simulink model "base"  (Simulink 7.2)
settings: Solver=FixedStepDiscrete  StartTime=0.0  StopTime=inf  FixedStep=0.001  RelTol=1e-3
PostLoadFcn:
  | , if any(exist('dsrtsu_mdlpostloadfcn', 'file') == [2, 3, 6]), try dsrtsu_mdlpostloadfcn('Execute', bdroot); catch fprintf('Error in PostLoadFcn (dsrtsu_mdlpostloadfcn) for model "%s":\n %s\n', bdroot, lasterr); end, end,
InitFcn:
  | DS4504_InitCallback(bdroot);
undefined symbols (not defined in the file or in its folder): IP, UDP
libraries: ds4504base_library x4, dsextras x1
settings Model: DSRTSU_INTERNAL_RTI_VER=340  DSRTSU_INTERNAL_RTI_TYPE=rti1005  Creator=yamakawa  LastModifiedBy=higo
settings OptimizationCC: BlockReduction=off  InlineInvariantSignals=on  InitFltsAndDblsToZero=on
settings DebuggingCC: SaveWithParameterizedLinksMsg=none  SignalResolutionControl=TryResolveAllWithWarning  MultiTaskDSMMsg=warning  MultiTaskCondExecSysMsg=none  StrictBusMsg=None
settings HardwareCC: ProdIntDivRoundTo=Zero  ProdEndianess=BigEndian  ProdHWDeviceType=Specified  TargetIntDivRoundTo=Zero  TargetEndianess=BigEndian
settings RTWCC: SystemTargetFile=rti1005.tlc  MakeCommand=make_rti  TemplateMakefile=rti1005.tmf  Description=dSPACE DS1005 Hardware Platform  ProcessScript=rti1005_make_rtw_hook  IncludeERTFirstTime=on
settings STFCustomTargetCC: TargetFcnLib=ansi_tfl_tmw.mat  SystemTargetFile=rti1005.tlc
settings GRTTargetCC: TargetFcnLib=ansi_tfl_tmw.mat  CompOptLevelCompliant=off  MatFileLogging=off  ExtModeMexFile=noextcomm
settings CustomProperty: DataType=RTWOptions_EnumType_C__dSPACE_matlab_rti1005_tlc_rti1005_InitialSimState  Value=STOP
settings EnumStrPairs: String=RUN

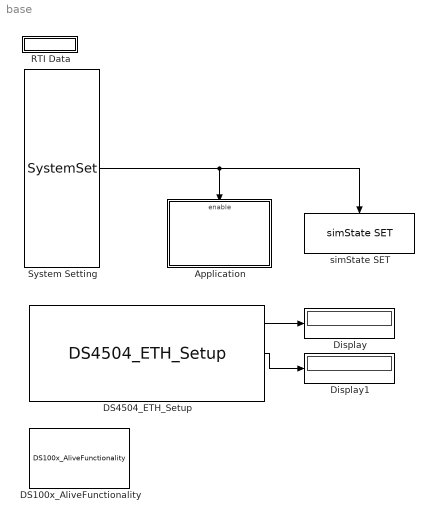
== system base ==
  Application : Subsystem  TreatAsAtomicUnit=on
  DS100x_AliveFunctionality : ds4504base_library/DS100x_AliveFunctionality  SystemSampleTime=-1  boardID=1
  DS4504_ETH_Setup : ds4504base_library/DS4504_ETH_Setup  boardID=1  IP=167888051  SM=4294901760  detectIP=off  numberApps=1  appTypes=1  appModes=1  generallyAcceptAnyIP=on  useChecksum=on  QNXSchedulerTimeInterval=50  receiveTimerPeriod=1  watchdogTimeoutSteps=10  rebootDS4504=on  DisplayMessages=on  ShowDialogBox=on  IP_String=10.1.196.179  warning1=on  warning2=on  warning3=on  warning4=on  warning5=on  disable_check=off
  Display : Display
  Display1 : Display
  RTI Data : Subsystem  Tag=struct('RTIDataServer',struct('RTIDataServerVs','2','RTIModelDescription','struct(''main'',''base'',''sub'','''',''isMp'',0)'))  LoadFcn="if exist('rtidc'), try,  rtidc('DataHostBlockClbLoad', gcbh); catch, disp(['Warning: ''LoadFcn'' for RTI Data block failed: ' lasterr]); end, end,"
      settings: CopyFcn="if exist('rtidc'), try,  rtidc('DataHostBlockClbCopy', gcbh); catch, disp(['Warning: ''CopyFcn'' for RTI Data block failed: ' lasterr]); end, end,"  DeleteFcn="if exist('rtidc'), try,  rtidc('DataHostBlockClbDelete', gcbh); catch, disp(['Warning: ''DeleteFcn'' for RTI Data block failed: ' lasterr]); end, end,"  ModelCloseFcn="if exist('rtidc'), try,  rtidc('DataHostBlockClbModelClose', gcbh); catch, disp(['Warning: ''ModelCloseFcn'' for RTI Data block failed: ' lasterr]); end, end,"  PreSaveFcn="if exist('rtidc'), try,  rtidc('DataHostBlockClbPreSave', gcbh); catch, disp(['Warning: ''PreSaveFcn'' for RTI Data block failed: ' lasterr]); end, end,"  PostSaveFcn="if exist('rtidc'), try,  rtidc('DataHostBlockClbPostSave', gcbh); catch, disp(['Warning: ''PostSaveFcn'' for RTI Data block failed: ' lasterr]); end, end,"  NameChangeFcn="if exist('rtidc'), try,  rtidc('DataHostBlockClbNameChange', gcbh); catch, disp(['Warning: ''NameChangeFcn'' for RTI Data block failed: ' lasterr]); end, end,"
      mask Type: RTI_DATA_HOST
      mask Description:
      | RTI Data Block.
      | This block is used by RTI to store internal model-dependent data.
      | Please keep this block on the root level of the model. Deleting this block will result in data loss.
      | 
      | NEVER DELETE OR COPY THIS BLOCK!
      mask Help:
      | RTI Data Block.
      | This block is used by RTI to store internal model-dependent data.
      | Please keep this block on the root level of the model. Deleting this block will result in data loss.
      | 
      | NEVER DELETE OR COPY THIS BLOCK!
      mask Display:
      | text(0.5, 0.5, 'RTI Data', 'HorizontalAlignment', 'center');
      | plot([1 0]);
  System Setting : S-Function  FunctionName=SystemSet  EnableBusSupport=off
  simState SET : dsextras/simState SET  SystemSampleTime=-1  TriggerPort=falling  EnablePort=none  SimStateMode=STOP  TLCFileName=rti_simstate_set  Reserved1=[]  Reserved2=[]  Reserved3=[]  Reserved4=[]  DSProperties=struct('RTI',struct('Version',uint32(1),'BlockType',struct('isSLSource',uint8(1),'isSLSink',uint8(0),'isHWSource',uint8(0),'isHWSink',uint8(0),'isSetup',uint8(0),'isInline',uint8(1),'isNonInline',uint8(0),'isInterrupt',uint8(0),'isChannelwise',uint8(0)),'IOBoardType','EXTRAS','UnitType','SIMSTATESET','Identifier','SIMSTATESET','DialogType','SL','BlockSet','NONE','SlaveProcessor','NONE'))  RTIBlockInterface=struct('OutputPortsWidth',int32(0),'BlockDisplay',{{['simState STOP'],'center'}},'IconTransparency','on','InitLevel',2,'BlockName',struct('Token',{{['simState SET']}}),'TriggerPort',{{'falling'}},'EnablePort',{{'none'}},'MaskDescription',['Set simState to the specified value when the block is executed.'])  RTIBlockParameters=struct('TriggerPort',{{3,'OFF',[]}},'EnablePort',{{1,'OFF',[]}},'SimStateMode',{{3,'OFF',[]}},'TLCFileName',{{'rti_simstate_set','OFF',[]}})  RTISFcnParameters=struct('TriggerPort','double','EnablePort','double','SimStateMode','char','TLCFileName','char')  RTIBlockParaDefault=struct('TriggerPort',2,'EnablePort',1,'SimStateMode',1,'TLCFileName','rti_simstate_set')
  wires:
  System Setting/1 -> Application/Enable, simState SET/Trigger
  DS4504_ETH_Setup/1 -> Display/1
  DS4504_ETH_Setup/2 -> Display1/1

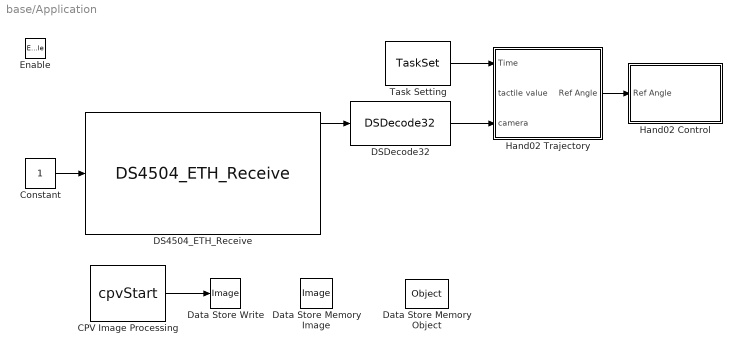
== system base/Application ==
  Enable : EnablePort  StatesWhenEnabling=reset
  CPV Image Processing : S-Function  FunctionName=cpvStart  EnableBusSupport=off
  Constant : Constant  OutDataType=sfix(16)  OutScaling=2^0
  DS4504_ETH_Receive : ds4504base_library/DS4504_ETH_Receive  boardID=1  IP1=10  IP2=1  IP3=196  IP4=179  IP=167888051  IP_String=10.1.196.179  acceptAnyIP=on  ethProtocol=UDP/IP  dynamicIPFiltering=off  receiveAsClient=off  TXConnectionPort=0  receivePort=50006  length=32  variableFrameLength=off  receiveMode=Sampling  queueSize=2048  sharePort=off  portSharingID=0  blockID=0
  "DSDecode32 " : ds4504base_library/DSDecode32   byteordering=little endian (Intel)  offset=[0]  auto_offset=on  datatype=9  one_datatype=on  sampletime=0.001
  Data Store Write : DataStoreWrite  DataStoreName=Image  SampleTime=-1
  Data Store Memory Image : DataStoreMemory  DataStoreName=Image  InitialValue=[-1 -1 0 0 0 0 0 0 0 0 0 0 0 0 0 0]  DataType=double  OutDataType=sfix(16)  OutScaling=2^0  OutDataTypeStr=double
  Data Store Memory Object : DataStoreMemory  DataStoreName=Object  InitialValue=[-1 0 0 0 0 0 0 0 0 0 0 0 0 0 0 0]  DataType=double  OutDataType=sfix(16)  OutScaling=2^0  OutDataTypeStr=double
  Hand02 Control : Subsystem
  Hand02 Trajectory : Subsystem
  Task Setting : S-Function  FunctionName=TaskSet  EnableBusSupport=off
  wires:
  Hand02 Trajectory/1(Ref Angle) -> Hand02 Control/1(Ref Angle)
  Task Setting/1 -> Hand02 Trajectory/1(Time)
  CPV Image Processing/1 -> Data Store Write/1
  Constant/1 -> DS4504_ETH_Receive/1
  "DSDecode32 "/1 -> Hand02 Trajectory/3(camera)
  DS4504_ETH_Receive/1 -> "DSDecode32 "/1

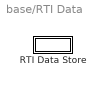
== system base/RTI Data ==
  RTI Data Store : Subsystem  Tag="struct('public',struct('sub',struct('name',{{'base'}},'data',{{struct('TH',struct('thTaskInfo',struct('taskType',{'TIMER','HWINT','TMRINT','SWINT'},'tasksNumOf',{1,0,0,0},'srcIds',{{'TIMERA'},{},{},{}},'taskNames',{{['Timer Task 1']},{},{},{}})),'th_tc',struct('dataType','TASK','taskGroupId','','taskGroupList',{{}},'taskSchedulingPolicy','FCFS','taskType','TIMER','blkh',-1,'srcId','TIMERA','srcSgnName',['Timer A interrupt'],'srcCpuName','','taskName',['Timer Task 1  [0.001] s'],'taskNameDisplayExt','','smplTime',0.001,'smplTimeOffs',0,'hasFixedPriority',0,'priority',1,'hasFixedOvc',0,'ovcType',1,'ovcMax',1),'tc_th',struct('dataType','TASK','taskGroupId','','taskGroupList',{{}},'taskSchedulingPolicy','FCFS','taskType','TIMER','blkh',-1,'srcId','TIMERA','srcSgnName',['Timer A interrupt'],'srcCpuName','','taskName',['Timer Task 1  [0.001] s'],'taskNameDisplayExt','','smplTime',0.001,'smplTimeOffs',0,'hasFixedPriority',0,'priority',1,'hasFixedOvc',0,'ovcType',1,'ovcMax',1))}})),'private',struct('version',struct('dsVer',uint32(2)),'access',struct('modified',['14-Dec-2017 23:02:08'],'type','Model','isPerm',1)))"
      mask Type: RTI_DATA_STORE
      mask Description:
      | RTI Data Store Block. This block is used by RTI to store internal model dependent data. Deleting this block will result in data loss.
      | 
      | NEVER DELETE, COPY, OR MODIFY THIS BLOCK!
      mask Help:
      | RTI Data Store Block. This block is used by RTI to store internal model dependent data. Deleting this block will result in data loss.
      | 
      | NEVER DELETE, COPY, OR MODIFY THIS BLOCK!
      mask Display: text(0.5, 0.5, ' ', 'HorizontalAlignment', 'center');

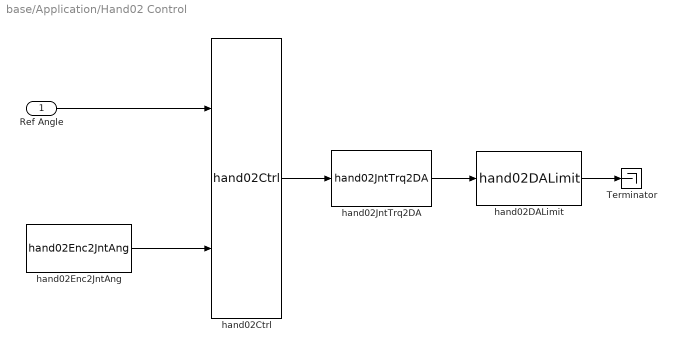
== system base/Application/Hand02 Control ==
  Ref Angle : Inport  OutDataType=sfix(16)  OutScaling=2^0
  Terminator : Terminator
  hand02Ctrl : S-Function  FunctionName=hand02Ctrl  EnableBusSupport=off
  hand02DALimit : S-Function  FunctionName=hand02DALimit  EnableBusSupport=off
  hand02Enc2JntAng : S-Function  FunctionName=hand02Enc2JntAng  EnableBusSupport=off
  hand02JntTrq2DA : S-Function  FunctionName=hand02JntTrq2DA  EnableBusSupport=off
  wires:
  Ref Angle/1 -> hand02Ctrl/1
  hand02Enc2JntAng/1 -> hand02Ctrl/2
  hand02Ctrl/1 -> hand02JntTrq2DA/1
  hand02JntTrq2DA/1 -> hand02DALimit/1
  hand02DALimit/1 -> Terminator/1

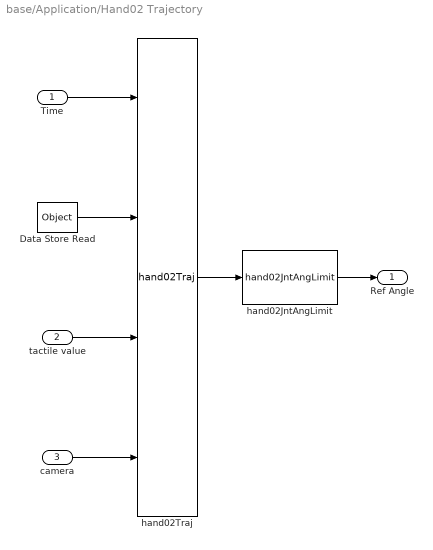
== system base/Application/Hand02 Trajectory ==
  Time : Inport  OutDataType=sfix(16)  OutScaling=2^0
  tactile value : Inport  Port=2  OutDataType=sfix(16)  OutScaling=2^0
  camera : Inport  Port=3  OutDataType=sfix(16)  OutScaling=2^0
  Data Store Read : DataStoreRead  DataStoreName=Object  SampleTime=0
  hand02JntAngLimit : S-Function  FunctionName=hand02JntAngLimit  EnableBusSupport=off
  hand02Traj : S-Function  FunctionName=hand02Traj  EnableBusSupport=off
  Ref Angle : Outport  OutDataType=sfix(16)  OutScaling=2^0
  wires:
  hand02Traj/1 -> hand02JntAngLimit/1
  Time/1 -> hand02Traj/1
  hand02JntAngLimit/1 -> Ref Angle/1
  Data Store Read/1 -> hand02Traj/2
  tactile value/1 -> hand02Traj/3
  camera/1 -> hand02Traj/4

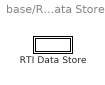
== system base/RTI Data/RTI Data Store ==
  RTI Data Store : Subsystem
      mask Type: RTI_DATA_STORE
      mask Description:
      | RTI Data Store Block. This block is used by RTI to store internal model dependent data. Deleting this block will result in data loss.
      | 
      | NEVER DELETE, COPY, OR MODIFY THIS BLOCK!
      mask Help:
      | RTI Data Store Block. This block is used by RTI to store internal model dependent data. Deleting this block will result in data loss.
      | 
      | NEVER DELETE, COPY, OR MODIFY THIS BLOCK!
      mask Display: text(0.5, 0.5, ' ', 'HorizontalAlignment', 'center');

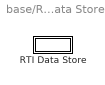
== system base/RTI Data/RTI Data Store/RTI Data Store ==
  RTI Data Store : Subsystem
      mask Type: RTI_DATA_STORE
      mask Description:
      | RTI Data Store Block. This block is used by RTI to store internal model dependent data. Deleting this block will result in data loss.
      | 
      | NEVER DELETE, COPY, OR MODIFY THIS BLOCK!
      mask Help:
      | RTI Data Store Block. This block is used by RTI to store internal model dependent data. Deleting this block will result in data loss.
      | 
      | NEVER DELETE, COPY, OR MODIFY THIS BLOCK!
      mask Display: text(0.5, 0.5, ' ', 'HorizontalAlignment', 'center');

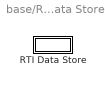
== system base/RTI Data/RTI Data Store/RTI Data Store/RTI Data Store ==
  RTI Data Store : Subsystem
      mask Type: RTI_DATA_STORE
      mask Description:
      | RTI Data Store Block. This block is used by RTI to store internal model dependent data. Deleting this block will result in data loss.
      | 
      | NEVER DELETE, COPY, OR MODIFY THIS BLOCK!
      mask Help:
      | RTI Data Store Block. This block is used by RTI to store internal model dependent data. Deleting this block will result in data loss.
      | 
      | NEVER DELETE, COPY, OR MODIFY THIS BLOCK!
      mask Display: text(0.5, 0.5, ' ', 'HorizontalAlignment', 'center');

== system base/RTI Data/RTI Data Store/RTI Data Store/RTI Data Store/RTI Data Store ==
